simulink model "Problem3"  (R2020b)
settings: Solver=VariableStepAuto  StartTime=0.0  StopTime=10  RelTol=1e-3
settings Model: Creator=HP  LastModifiedBy=HP

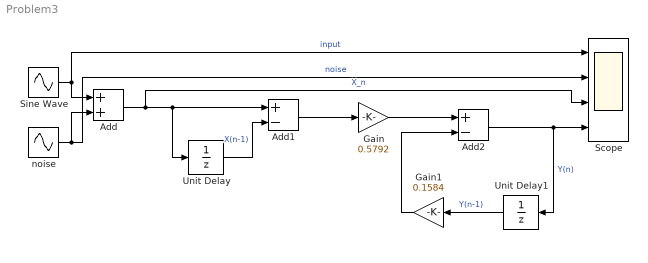
== system Problem3 ==
  Add : Sum
  Add1 : Sum  Inputs=+-
  Add2 : Sum  Inputs=+-
  Gain : Gain  Gain=0.5792
  Gain1 : Gain  Gain=0.1584
  Scope : Scope  NumInputPorts=4
  Sine Wave : Sin  Frequency=100  SampleTime=0
  Unit Delay : UnitDelay  SampleTime=-1  HasFrameUpgradeWarning=on
  Unit Delay1 : UnitDelay  SampleTime=-1  HasFrameUpgradeWarning=on
  noise : Sin  Amplitude=0.5  SampleTime=0
  wires:
  Sine Wave/1 -> Add/1, Scope/1  "input"
  noise/1 -> Scope/2, Add/2  "noise"
  Add/1 -> Scope/3, Add1/1, Unit Delay/1  "X_n"
  Unit Delay/1 -> Add1/2  "X(n-1)"
  Add1/1 -> Gain/1
  Gain/1 -> Add2/1
  Add2/1 -> Unit Delay1/1, Scope/4  "Y(n)"
  Gain1/1 -> Add2/2
  Unit Delay1/1 -> Gain1/1  "Y(n-1)"
